simulink model "Exercise_4"  (R2020b)
settings: Solver=VariableStepAuto  StartTime=0.0  StopTime=0.1  RelTol=1e-3
libraries: powerlib x9, powerlib_meascontrol x2
settings Model: Creator=ADMIN  LastModifiedBy=macbook
settings SFSimCC: CustomCodeUndefinedFunction=UseInterfaceOnly

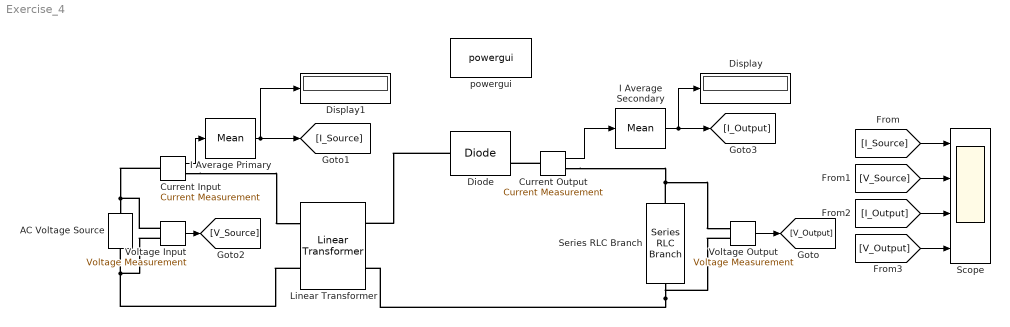
== system Exercise_4 ==
  AC Voltage Source : powerlib/Electrical Sources/AC Voltage Source  Amplitude=339.41  Phase=0  Frequency=60  SampleTime=0  Measurements=None  BusType=swing  Pref=10e3  Qref=0  Qmin=-inf  Qmax=+inf
  Current Input : powerlib/Measurements/Current Measurement  PhasorSimulation=off  OutputType=Complex  PSBequivalent=0
  Current Output : powerlib/Measurements/Current Measurement  PhasorSimulation=off  OutputType=Complex  PSBequivalent=0
  Diode : powerlib/Power Electronics/Diode  Ron=0.001  Lon=0  Vf=0.6  IC=0  UseSnubber=0  Rs=0  Cs=0  Measurements=on
  Display : Display
  Display1 : Display
  I Average Primary : powerlib_meascontrol/Measurements/Mean  Freq=60  Vinit=0  Ts=0
  I Average Secondary : powerlib_meascontrol/Measurements/Mean  Freq=60  Vinit=0  Ts=0
  Linear Transformer : powerlib/Elements/Linear Transformer  UNITS=pu  NominalPower=[ 250e6 60 ]  winding1="[ 240  0.002  0.08 ]"  winding2="[ 532.88  0.002  0.08 ]"  ThreeWindings=off  winding3=[ 315e3 0.002 0.08 ]  RmLm=[ 500 500 ]  Measurements=None  DataType=off
  Scope : Scope  NumInputPorts=4
  Series RLC Branch : powerlib/Elements/Series RLC Branch  LConnTagsString=__new0  RConnTagsString=__new0  BranchType=R  Resistance=20  Inductance=1e-3  SetiL0=off  InitialCurrent=0  Capacitance=1e-6  Setx0=off  InitialVoltage=0  Measurements=None
  Voltage Input : powerlib/Measurements/Voltage Measurement  PhasorSimulation=off  OutputType=Complex  PSBequivalent=0
  Voltage Output : powerlib/Measurements/Voltage Measurement  PhasorSimulation=off  OutputType=Complex  PSBequivalent=0
  powergui : powerlib/powergui  Priority=1  SimulationMode=Continuous  SampleTime=50e-6  frequency=60  Iterations=50  frequencyindice=60  Pbase=100e6  ErrMax=1e-4  UnitsV=kV  UnitsW=MW  buscounter=0  FunctionMessages=off  echomessages=off  EnableUseOfTLC=off  CurrentSourceSwitches=off  DisableSnubberDevices=off  DisableRonSwitches=off  DisableVfSwitches=off  DisplayEquations=off  AutomaticDiscreteSolvers=off  SolverType=Tustin/Backward Euler (TBE)  Interpol=off  ExternalGateDelay=off  methode=off  Ts=100  x0status=blocks  SPID=on  SwTol=0  HookPort=off  NonlinearTolerance=0  nMaxIteration=15  ContinueOnMaxIteration=off  RestoreLinks=warning  ResistiveCurrentMeasurement=off  Frange=[0:2:500]  Ylog=off  Xlog=on  ShowGrid=off  save=off  variable=ZData  structure=0  ZoomFFT=off  StartTime=0.0  cycles=1  DisplayStyle=1  fundamental=60  FreqAxis=off  MaxFrequency=1000  frequencyindicesteady=1  RmsSteady=1  display=off
  wires:
  Voltage Input/1 -> [V_Source]
  Voltage Output/1 -> [V_Output]
  [V_Output] -> Scope/4
  [I_Output] -> Scope/3
  [V_Source] -> Scope/2
  [I_Source] -> Scope/1
  I Average Secondary/1 -> Display/1, [I_Output]
  Current Output/1 -> I Average Secondary/1
  I Average Primary/1 -> Display1/1, [I_Source]
  Current Input/1 -> I Average Primary/1
  connections:
  Current Input/LConn1 -- Voltage Input/LConn1 -- AC Voltage Source/RConn1
  Current Input/RConn1 -- Linear Transformer/LConn1
  Linear Transformer/LConn2 -- AC Voltage Source/LConn1 -- Voltage Input/LConn2
  Current Output/LConn1 -- Diode/RConn1
  Diode/LConn1 -- Linear Transformer/RConn1
  Series RLC Branch/RConn1 -- Linear Transformer/RConn2 -- Voltage Output/LConn2
  Series RLC Branch/LConn1 -- Current Output/RConn1 -- Voltage Output/LConn1
